simulink model "ControlDes"  (R2026a)
settings: Solver=ode3  StopTime=4  FixedStep=0.001  EnableMultiTasking=on
(part 4 of 12)

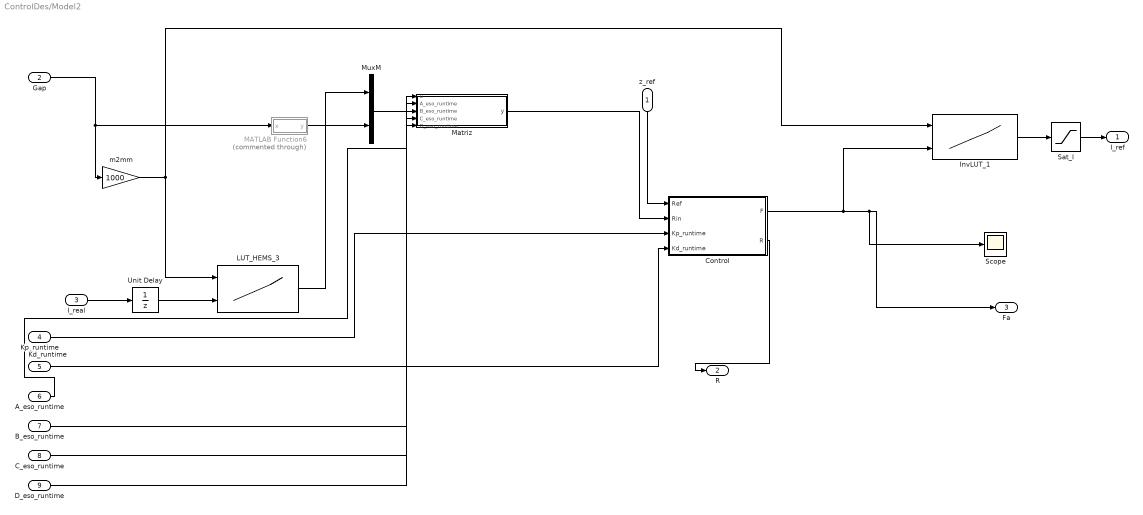
== system ControlDes/Model2 ==
  z_ref : Inport
  Gap : Inport  Port=2
  I_real : Inport  Port=3
  Kp_runtime : Inport  Port=4  OutDataTypeStr=double
  Kd_runtime : Inport  Port=5  OutDataTypeStr=double
  A_eso_runtime : Inport  Port=6  OutDataTypeStr=double  PortDimensions=[3 3]
  B_eso_runtime : Inport  Port=7  OutDataTypeStr=double  PortDimensions=[3 2]
  C_eso_runtime : Inport  Port=8  OutDataTypeStr=double  PortDimensions=[3 3]
  D_eso_runtime : Inport  Port=9  OutDataTypeStr=double  PortDimensions=[3 2]
  Control : Subsystem
  InvLUT_1 : Lookup_n-D  BreakpointsForDimension1=[4 4.5 5 5.5 6 6.5 7 7.5 8 8.5 9 9.5 10 10.5 11 11.5 12 12.5 13 13.5 14 14.5 15 15.5 16 16.5 17 17.5 18 18.5 19 19.5 20 20.5 21 21.5 22]  BreakpointsForDimension2=[47.107942170000001 66.738994842512568 86.370047515025135 106.00110018753769 125.63215286005025 145.26320553256284 164.89425820507537 184.52531087758794 204.15636355010051 223.78741622261307 243.41846889512564 263.04952156763818 282.68057424015075 302.31162691266331 321.94267958517588 341.57373225768845 361.20478493020101 380.83583760271358 400.46689027522615 420.09794294773872 439.72899562025128 459.36004829276385 478.99110096527642 498.62215363778898 518.25320631030149 537.88425898281412 557.51531165532663 577.14636432783925 596.77741700035176 616.40846967286438 636.03952234537689 655.67057501788952 675.30162769040203 694.93268036291454 714.56373303542716 734.19478570793967 753.8258383804523 773.45689105296481 793.08794372547743 812.71899639798994 832.35004907050256 851.98110174301507 871.6121544155277 891.24320708804021 910.87425976055283 930.50531243306534 950.13636510557797 969.76741777809048 989.39847045060299 1009.0295231231156 1028.6605757956281 1048.2916284681407 1067.9226811406534 1087.5537338131658 1107.1847864856786 1126.815839158191 1146.4468918307034 1166.0779445032163 1185.7089971757287 1205.3400498482411 1224.9711025207539 1244.6021551932663 1264.2332078657791 1283.8642605382915 1303.4953132108039 1323.1263658833168 1342.7574185558292 1362.3884712283416 1382.0195239008544 1401.6505765733668 1421.2816292458792 1440.9126819183921 1460.5437345909045 1480.1747872634173 1499.8058399359297 1519.4368926084421 1539.067945280955 1558.6989979534674 1578.3300506259798 1597.9611032984926 1617.592155971005 1637.2232086435174 1656.8542613160303 1676.4853139885427 1696.1163666610555 1715.7474193335679 1735.3784720060803 1755.0095246785932 1774.6405773511055 1794.2716300236179 1813.9026826961308 1833.5337353686432 1853.164788041156 1872.7958407136684 1892.4268933861808 1912.0579460586937 1931.6889987312061 1951.3200514037185 1970.9511040762313 1990.5821567487437 2010.2132094212561 2029.844262093769 2049.4753147662814 2069.1063674387942 2088.7374201113066 2108.3684727838195 2127.9995254563319 2147.6305781288443 2167.2616308013571 2186.8926834738695 2206.5237361463819 2226.1547888188948 2245.7858414914072 2265.4168941639196 2285.0479468364324 2304.6789995089448 2324.3100521814576 2343.94110485397 2363.5721575264824 2383.2032101989953 2402.8342628715077 2422.4653155440201 2442.0963682165329 2461.7274208890453 2481.3584735615582 2500.9895262340706 2520.620578906583 2540.2516315790958 2559.8826842516082 2579.5137369241206 2599.1447895966335 2618.7758422691459 2638.4068949416583 2658.0379476141711 2677.6690002866835 2697.3000529591964 2716.9311056317088 2736.5621583042212 2756.193210976734 2775.8242636492464 2795.4553163217588 2815.0863689942717 2834.717421666784 2854.3484743392969 2873.9795270118093 2893.6105796843217 2913.2416323568345 2932.8726850293469 2952.5037377018593 2972.1347903743722 2991.7658430468846 3011.396895719397 3031.0279483919098 3050.6590010644222 3070.2900537369351 3089.9211064094475 3109.5521590819599 3129.1832117544727 3148.8142644269851 3168.4453170994975 3188.0763697720104 3207.7074224445228 3227.3384751170352 3246.969527789548 3266.6005804620604 3286.2316331345733 3305.8626858070857 3325.4937384795981 3345.1247911521109 3364.7558438246233 3384.3868964971357 3404.0179491696485 3423.6490018421609 3443.2800545146738 3462.9111071871862 3482.5421598596986 3502.1732125322114 3521.8042652047238 3541.4353178772362 3561.0663705497491 3580.6974232222615 3600.3284758947739 3619.9595285672867 3639.5905812397991 3659.221633912312 3678.8526865848244 3698.4837392573368 3718.1147919298496 3737.745844602362 3757.3768972748744 3777.0079499473873 3796.6390026198997 3816.2700552924121 3835.9011079649249 3855.5321606374373 3875.1632133099502 3894.7942659824625 3914.4253186549749 3934.0563713274878 3953.6874240000002]  Table=[-55 -55 -55 -55 -55 -55 -55 -55 -55 -55 -55 -55 -55 -55 -55 -55 -55 -55 -55 -55 -55 -55 -55 -55 -55 -55 -55 -55 -55 -55 -55 -55 -55 -55 -54.432628320800852 -53.430146611134205 -52.45463633914374 -51.503874127967528 -50.576822658402456 -49.671150181099165 -48.785244676788871 -47.917749917322467 -47.06811189824262 -46.23545295987752 -45.417695369856638 -44.625186259027025 -43.826690201682588 -43.050940103614955 -42.301872770566156 -41.552121023695143 -40.803731049854143 -40.08126794385975 -39.355489875938929 -38.657187874569566 -37.956411551237629 -37.254788106526306 -36.572472365677079 -35.915261986845785 -35.238731215369704 -34.582140705771778 -33.933419958233905 -33.298597326241975 -32.672759517500708 -32.030580694488748 -31.420081201769687 -30.794491157978158 -30.18325123394094 -29.579556424548343 -28.981492025551898 -28.390394280497176 -27.802385700901638 -27.219822635876184 -26.642972491511646 -26.069215047149669 -25.504624250761417 -24.940052662110087 -24.375242750913273 -23.816965375934146 -23.265863070195717 -22.717038456749641 -22.169576845090784 -21.613454968077011 -21.063779832162339 -20.522907043508095 -19.983167877750141 -19.445751525511753 -18.913238727901682 -18.393182280250361 -17.895187218822535 -17.368108519503462 -16.835998655338848 -16.306000754109316 -15.778571842608143 -15.253668812040141 -14.731610349826674 -14.212095847002193 -13.694973083562758 -13.174151558087285 -12.648608531780747 -12.122916991641022 -11.598969181622328 -11.077165220210059 -10.557040236805376 -10.039158527890619 -9.5234046996748187 -9.010000704832084 -8.4942364433276509 -7.9734520616161761 -7.4532619117384895 -6.9338696328660543 -6.4153825023130668 -5.8988123034756628 -5.3841268352005764 -4.8706064982437605 -4.3588297827106217 -3.848316029612564 -3.3369297227567936 -2.8224661401082973 -2.3074711937118657 -1.7927557158394691 -1.2788850771910441 -0.76575900337409364 -0.25314382340547825 0.26471705934941686 0.8306291619239724 1.4464597395275431 2.0768002565023478 2.714498666138367 3.3575913116100984 4.0058073222110702 4.6557755139368426 5.3082747450239625 5.9624210174100787 6.6160889098987363 7.2697049106362535 7.9269522692399574 8.5890540478063873 9.2507801960733271 9.9124794262809779 10.574952848078006 11.237938887511772 11.901766174713323 12.566027053477136 13.230907075578958 13.897816482644709 14.570346157163394 15.246664657432234 15.921413279630494 16.608755968667605 17.303668261070609 18.004386174276554 18.706276444844143 19.407993677187967 20.113713425365059 20.821720378182569 21.53228186213769 22.250085832108567 22.972548319358236 23.695843569924715 24.4269351104797 25.170690797556379 25.918303156235122 26.669208444309753 27.424510923793964 28.183818112160029 28.945437687541883 29.711125199052763 30.477484186499211 31.244135976555402 32.010572523951964 32.776356224193975 33.541812324131911 34.307576697883754 35.073398028271967 35.8397080862525 36.606723723928724 37.372699542527002 38.139657308160615 38.906516058624483 39.673024301960652 40.438516430531017 41.203427642119735 41.967823824632816 42.734415506477788 43.501091277007703 44.266162855242563 45.034670730785479 45.801611239709203 46.567861396973932 47.334851296139263 48.099285442923062 48.867255985870152 49.634194962270875 50.400860404303749 51.166964635064488 51.931664668231846 52.698534187926221 53.466323409936088 54.232657391262379 55;-55 -55 -55 -55 -55 -55 -55 -55 -55 -55 -55 -55 -55 -55 -55 -55 -55 -55 -55 -55 -55 -55 -55 -55 -55 -55 -55 -55 -55 -55 -55 -54.277257681775673 -53.213703712619242 -52.180445920815295 -51.175176457963069 -50.195665817912335 -49.239950921593476 -48.306290430535796 -47.393166249606459 -46.499149156938124 -45.624301835043788 -44.76612693392066 -43.923587859320996 -43.096730138152708 -42.284444361967736 -41.4849798974085 -40.699600135100638 -39.933738377860266 -39.164322887957262 -38.427573249819034 -37.679652777812606 -36.956634665628428 -36.224779239470536 -35.525923184948347 -34.824246868106989 -34.12347391991829 -33.436940003991509 ...(+73925 chars)]  ExtrapMethod=Clip  InternalRulePriority=Speed  RndMeth=Simplest
      settings: InputPortMap=u0,u1
  LUT_HEMS_3 : Lookup_n-D  BreakpointsForDimension1=[4 4.5 5 5.5 6 6.5 7 7.5 8 8.5 9 9.5 10 10.5 11 11.5 12 12.5 13 13.5 14 14.5 15 15.5 16 16.5 17 17.5 18 18.5 19 19.5 20 20.5 21 21.5 22]  BreakpointsForDimension2=[-55 -54.5 -54 -53.5 -53 -52.5 -52 -51.5 -51 -50.5 -50 -49.5 -49 -48.5 -48 -47.5 -47 -46.5 -46 -45.5 -45 -44.5 -44 -43.5 -43 -42.5 -42 -41.5 -41 -40.5 -40 -39.5 -39 -38.5 -38 -37.5 -37 -36.5 -36 -35.5 -35 -34.5 -34 -33.5 -33 -32.5 -32 -31.5 -31 -30.5 -30 -29.5 -29 -28.5 -28 -27.5 -27 -26.5 -26 -25.5 -25 -24.5 -24 -23.5 -23 -22.5 -22 -21.5 -21 -20.5 -20 -19.5 -19 -18.5 -18 -17.5 -17 -16.5 -16 -15.5 -15 -14.5 -14 -13.5 -13 -12.5 -12 -11.5 -11 -10.5 -10 -9.5 -9 -8.5 -8 -7.5 -7 -6.5 -6 -5.5 -5 -4.5 -4 -3.5 -3 -2.5 -2 -1.5 -1 -0.5 0 0.5 1 1.5 2 2.5 3 3.5 4 4.5 5 5.5 6 6.5 7 7.5 8 8.5 9 9.5 10 10.5 11 11.5 12 12.5 13 13.5 14 14.5 15 15.5 16 16.5 17 17.5 18 18.5 19 19.5 20 20.5 21 21.5 22 22.5 23 23.5 24 24.5 25 25.5 26 26.5 27 27.5 28 28.5 29 29.5 30 30.5 31 31.5 32 32.5 33 33.5 34 34.5 35 35.5 36 36.5 37 37.5 38 38.5 39 39.5 40 40.5 41 41.5 42 42.5 43 43.5 44 44.5 45 45.5 46 46.5 47 47.5 48 48.5 49 49.5 50 50.5 51 51.5 52 52.5 53 53.5 54 54.5 55]  Table=[703.68896489999997 713.25615619999996 722.96035870000003 732.80062650000002 742.77980739999998 752.8957001 763.14771970000004 773.53739289999999 784.06407369999999 794.72611670000003 805.5261041 816.4625436 827.53520409999999 838.74527539999997 850.09215349999999 861.57511 873.19506939999997 884.95113779999997 896.8432937 908.87169949999998 921.03723779999996 933.66761069999995 945.77772600000003 958.35243079999998 971.06230210000001 984.16869589999999 997.36671660000002 1010.386759 1023.258554 1037.020338 1050.4791720000001 1063.8307789999999 1077.9886180000001 1091.9395770000001 1105.9790640000001 1119.8098210000001 1134.095462 1148.540645 1163.6569010000001 1177.942364 1192.8056650000001 1207.803997 1222.9380389999999 1238.205854 1254.085239 1269.590608 1284.7941290000001 1300.9965970000001 1316.629441 1332.4363639999999 1348.7285420000001 1364.9732059999999 1381.405321 1397.998247 1414.659465 1431.414741 1448.364613 1465.4208920000001 1482.5453239999999 1499.966964 1517.3595700000001 1534.6857990000001 1552.2484910000001 1569.8694929999999 1587.9370349999999 1605.6498099999999 1623.7211010000001 1641.1862169999999 1659.1450890000001 1677.317884 1695.502035 1713.7508230000001 1732.1531500000001 1750.740487 1770.723303 1789.41031 1807.8395519999999 1826.3245549999999 1844.9049889999999 1863.5561829999999 1882.3107259999999 1901.156772 1920.088722 1939.103891 1957.849048 1976.4921529999999 1995.1750469999999 2013.924432 2032.7495510000001 2051.6291030000002 2070.5914419999999 2089.6285349999998 2108.7509479999999 2127.782279 2146.6288410000002 2165.4954120000002 2184.3902670000002 2203.3105949999999 2222.2968639999999 2241.3600750000001 2260.4575359999999 2279.6213969999999 2298.8412790000002 2318.0843159999999 2337.173436 2356.2336559999999 2375.291847 2394.3788949999998 2413.498744 2432.6383729999998 2451.795267 2470.55521 2486.8926430000001 2502.6800499999999 2518.2489300000002 2533.6893009999999 2548.9862039999998 2564.2221450000002 2579.3381850000001 2594.45289 2609.5127010000001 2624.5368659999999 2639.5340529999999 2654.5471259999999 2669.5822469999998 2684.5741010000002 2699.4773500000001 2714.289585 2729.120582 2743.9574320000002 2758.7894190000002 2773.6024739999998 2788.4237229999999 2803.1997719999999 2817.9927010000001 2832.7675509999999 2847.533246 2862.290759 2876.9819149999998 2891.5663249999998 2906.0962920000002 2920.5802079999999 2935.1650319999999 2949.4169959999999 2963.6081330000002 2977.6475610000002 2991.643204 3005.623388 3019.617976 3033.6010019999999 3047.4952549999998 3061.4063040000001 3075.2129359999999 3089.0343520000001 3102.7689129999999 3116.3307490000002 3129.9298480000002 3143.5074070000001 3157.056122 3170.3944430000001 3183.58106 3196.7490509999998 3209.847651 3222.927013 3235.9625980000001 3248.9268459999998 3261.850312 3274.7714230000001 3287.6354110000002 3300.453548 3313.263809 3326.0704420000002 3338.874292 3351.6755579999999 3364.4850160000001 3377.2931130000002 3390.1276050000001 3402.9466910000001 3415.7570070000002 3428.586319 3441.400682 3454.2032909999998 3467.0199069999999 3479.8068020000001 3492.6219369999999 3505.4355770000002 3518.2302589999999 3531.0258880000001 3543.8291089999998 3556.6326370000002 3569.4450959999999 3582.275091 3595.105579 3607.942814 3620.7860190000001 3633.597182 3646.3808909999998 3659.1935640000002 3672.054603 3684.8251369999998 3697.5946680000002 3710.4163079999998 3723.1785709999999 3736.0069319999998 3748.8191689999999 3761.5975699999999 3774.4683279999999 3787.257826 3800.0298120000002 3812.8328069999998 3825.6397270000002 3838.4389219999998 3851.2470440000002 3864.0794519999999 3876.9178449999999 3889.7194530000002 3902.5001560000001 3915.286521 3928.0923950000001 3940.909474 3953.6874240000002;642.64808679999999 651.6175958 660.715506 669.94350099999997 679.30116109999994 688.78706220000004 698.40299040000002 708.14882739999996 718.02327430000003 728.02695159999996 738.1602762 748.42185340000003 758.81217089999996 769.33143840000002 ...(+135712 chars)]  ExtrapMethod=Clip  InternalRulePriority=Speed  RndMeth=Simplest
      settings: InputPortMap=u0,u1
  MATLAB Function6 : MATLAB Function  Commented=through  TreatAsAtomicUnit=on
  Matriz : Subsystem
  MuxM : Mux  Inputs=2
  Sat_I : Saturate  UpperLimit=50  LowerLimit=-50
  Scope : Scope
      settings: ActiveDisplayYMinimum=-11967.729581091611  ActiveDisplayYMaximum=16975.635504075348  DataLoggingVariableName=ScopeData2
  Unit Delay : UnitDelay  SampleTime=-1
  m2mm : Gain  Gain=1000
  I_ref : Outport
  R : Outport  Port=2
  Fa : Outport  Port=3
  wires:
  LUT_HEMS_3/1 -> MuxM/1
  Sat_I/1 -> I_ref/1
  InvLUT_1/1 -> Sat_I/1
  Unit Delay/1 -> LUT_HEMS_3/2
  m2mm/1 -> InvLUT_1/1, LUT_HEMS_3/1
  Gap/1 -> m2mm/1, MATLAB Function6/1(x)
  I_real/1 -> Unit Delay/1
  MuxM/1 -> Matriz/1(u)
  z_ref/1 -> Control/1(Ref)
  Matriz/1(y) -> Control/2(Rin)
  Control/1(F) -> InvLUT_1/2, Scope/1, Fa/1
  Control/2(R) -> R/1
  MATLAB Function6/1(y) -> MuxM/2
  Kp_runtime/1 -> Control/3(Kp_runtime)
  Kd_runtime/1 -> Control/4(Kd_runtime)
  A_eso_runtime/1 -> Matriz/2(A_eso_runtime)
  B_eso_runtime/1 -> Matriz/3(B_eso_runtime)
  C_eso_runtime/1 -> Matriz/4(C_eso_runtime)
  D_eso_runtime/1 -> Matriz/5(D_eso_runtime)
